simulink subsystem "MotorDriveGearTh"  (R2024b)
settings: Solver=VariableStepAuto  StartTime=0.0  StopTime=10.0  RelTol=1e-3
model mask{max_torque=electricDrive.max_torque, max_power=electricDrive.max_power, Tctc=electricDrive.Tctc, motor_loss_map=electricDrive.motor_loss_map, coolant_channel_D=electricDrive.coolant_channel_D}
  mask prompts: Tctc "Motor torque control time constant(s)"; coolant_channel_D "[m] Coolant jacket channels diameter"
undefined symbols (not defined in the file or in its folder): electricDrive, vehicleThermal
libraries: fl_lib x20, ee_lib x4, SimscapeFluids_lib x2, nesl_utility x2, EmotorLib x1, sdl_lib x1
Description:
  | Motor Drive with Gear (Thermal)
  | 
  | ⚡ Main Features:
  | - Electric motor model coupled with fixed gear
  | - Motor input interface: torque command, battery signals, and control
  | - Includes motor plant with electrical, mechanical, and thermal ports
  | - Coolant jacket for motor thermal management
  | - Inverter thermal dynamics with coolant pipe connection
  | - Gear block transmits torque to axle
  | 
  | 📤 Outputs: Motor Torque, Motor Speed, Electrical Power, Thermal States, Energy
  | 
  | 📌 Use Case: Powertrain simulations with electro-mechanical coupling and thermal effects
settings Model: Creator=jjha  LastModifiedBy=jjha

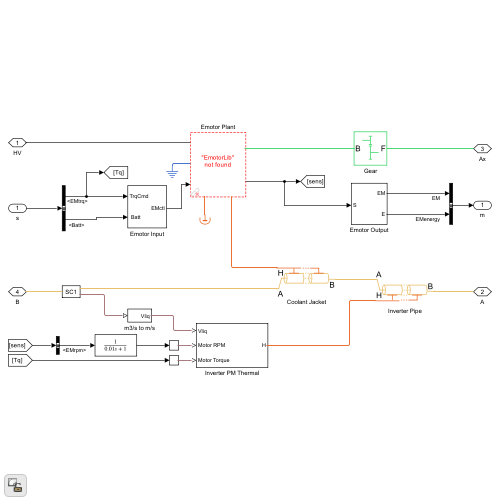
[thumbnail: Simulink's stored preview of the top-level diagram]
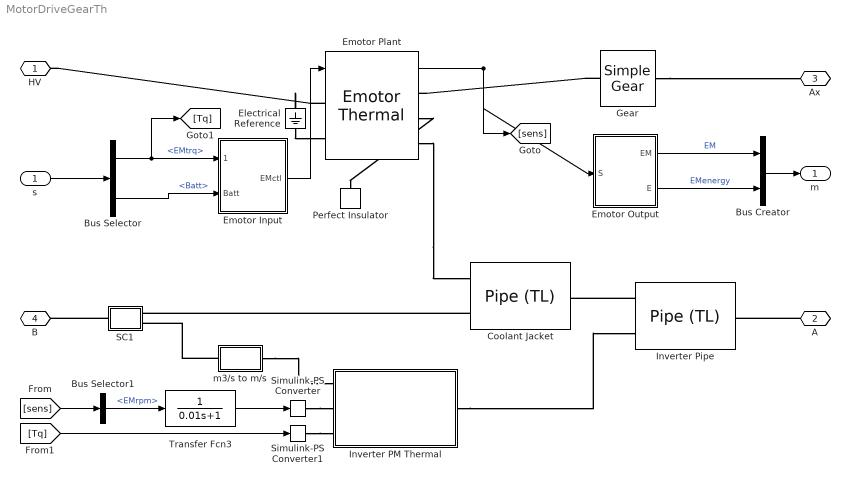
== system MotorDriveGearTh ==
  s : Inport
  Bus Creator : BusCreator  Inputs=2
  Bus Selector : BusSelector  OutputSignals=EMtrq,Batt
  Bus Selector1 : BusSelector  OutputSignals=EMrpm
  Coolant Jacket : SimscapeFluids_lib/Thermal Liquid/Pipes & Fittings/Pipe (TL)  dynamic_compressibility=false  inertia=0  num_segments=1  pipe_length=0.4 m  cross_section_geometry=fluids.thermal_liquid.pipes_fittings.enum.CrossSectionGeometry.Custom  pipe_diameter=0.1 m  pipe_inner_diameter=0.05 m  pipe_outer_diameter=0.1 m  pipe_width=0.1 m  pipe_height=0.1 m  pipe_major_axis=0.1 m  pipe_minor_axis=0.05 m  pipe_side=0.1 m  pipe_angle=30 deg  area=4 * pi * electricDrive.coolant_channel_D^2 / 4 m^2  Dh=electricDrive.coolant_channel_D m  elevation_spec=foundation.enum.constant_variable.constant  elevation_gain=0 m  gravity_spec=foundation.enum.constant_variable.constant  g=9.81 m/s^2  pressure_loss_spec=1  local_pressure_loss_spec=fluids.thermal_liquid.pipes_fittings.enum.LocalLossSpec.AggregateLength  length_add=20 * electricDrive.coolant_channel_D * 4 m  loss_coefficient=0.1  roughness_spec=fluids.thermal_liquid.pipes_fittings.enum.RoughnessSpec.Custom  roughness=1.5e-5 m  Re_friction_TLU=[ 400 1000 1.5e+3 3e+3 4e+3 6e+3 1e+4 2e+4 4e+4 6e+4 1e+5 1e+8 ]  friction_factor_TLU=[ 0.264 0.112 0.07099999999999999 0.0417 0.0387 0.0268 0.025 0.0232 0.0226 0.022 0.0214 0.0214 ]  Re_lam=100  Re_tur=500  shape_factor=64  mdot_nominal=[ 0.1 1 ] kg/s  p_diff_nominal=[ 0.001 0.01 ] MPa  mdot_threshold=1e-6 kg/s  wall_spec=1  vol_expansion_spec=fluids.thermal_liquid.pipes_fittings.enum.VolumeExpansionSpec.Diameter  area_pressure_gain=1e-6 m^2/MPa  static_pressure_TLU=[.1, 1] MPa  area_pressure_gain_TLU=[1e-05, 1.1e-05] m^2  material_behavior_spec=fluids.thermal_liquid.pipes_fittings.enum.PipeMaterialBehavior.Linear  diameter_pressure_gain=1.2e-6 m/MPa  wall_thickness=0.05 m  elastic_modulus=69 GPa  stress_TLU=[276, 310] MPa  strain_TLU=[.004, .02]  stress_assert_action=simscape.enum.assert.action.none  stress_max=400 MPa  poisson_ratio=0.33  wall_time_constant=0.01 s  thermal_expansion=false  alpha_L_wall=24 um/(deltaK*m)  thermal_expansion_Tref=293.15 K  heat_transfer_spec=4  mdot_nominal_heat=[ 0.1 1 ] kg/s  T_in_nominal=[ 293.15 293.15 ] K  T_out_nominal=[ 300 300 ] K  p_in_nominal_heat=[ 0.101325 0.101325 ] MPa  T_wall_nominal=[ 303.15 303.15 ] K  a_coeff=0.3  b_Re_power=0.8  c_Pr_power=0.33  Nu_lam=3.66  Re_Colburn_TLU=[ 100 150 1000 ]  Colburn_factor_TLU=[ 0.019 0.013 0.002 ]  Re_Nu_TLU=[ 100 150 1000 ]  Pr_Nu_TLU=[ 1 10 ]  Nu_TLU=[ 3.72 4.21; 3.75 4.44; 4.21 7.15 ]  p0_vec=vehicleThermal.coolant_p_init MPa  T0_vec=vehicleThermal.coolant_T_init K  mdot0=0.1 kg/s
  Electrical Reference : fl_lib/Electrical/Electrical Elements/Electrical Reference
  Emotor Input : Subsystem
  Emotor Output : Subsystem
  Emotor Plant : EmotorLib/Emotor Thermal  InitTemp=vehicleThermal.coolant_T_init  IronSpHeat=electricDrive.IronSpHeat  CopperSpHeat=electricDrive.CopperSpHeat  IronThConductivity=electricDrive.IronThConductivity  GrossToothMass=electricDrive.MotorThermal.GrossToothMass  WindingMass=electricDrive.MotorThermal.WindingMass  max_torque=electricDrive.max_torque  max_power=electricDrive.max_power  Tctc=electricDrive.Tctc  spMat=electricDrive.motor_loss_map.spMat  tqMat=electricDrive.motor_loss_map.tqMat  lossMat=electricDrive.motor_loss_map.lossMat  StatorBackIronMass=electricDrive.MotorThermal.StatorBackIronMass  StatorRootDia=electricDrive.MotorThermal.StatorRootDia  stator_od=electricDrive.MotorThermal.stator_od  StatorWindingOhArea=electricDrive.MotorThermal.StatorWindingOhArea  Bridgemass=electricDrive.MotorThermal.Bridgemass  rotor_od=electricDrive.MotorThermal.rotor_od  rotorStackLength=electricDrive.MotorThermal.rotorStackLength  RotorBackIronMass=electricDrive.MotorThermal.RotorBackIronMass  RotorAreaER=electricDrive.MotorThermal.RotorAreaER  RotorAreaCyl=electricDrive.MotorThermal.RotorAreaCyl
  Gear : sdl_lib/Gears/Simple Gear  ratio=10/3  rotation_direction=sdl.enum.shaftOutputDirection.same  friction_model=sdl.enum.gear_efficiencies_load.off  T_noload=0.1 N*m  T_nom=5 N*m  efficiency_nom=0.8  efficiency=0.8  temperature_TLU=[280, 300, 320] K  load_TLU=[1, 5, 10] N*m  efficiency_TLU=[.95, .9, .85]  efficiency_TLU2=[.85, .8, .75; .95, .9, .85; .85, .8, .7]  w_thr=0.01 rad/s  pwr_thr=0.001 W  enable_backlash=false  hardstop_model=simscape.enum.hardstop.smooth  backlash_distance=1e-3 mm  r_base=0.1 m  transition=1e-4 mm  backlash_stiffness=1e7 N/m  backlash_damping=1e6 N*s/m  coeff_rest=0  v_tol=0.001 m/s  f_tol=0 N  mu_visc=[0, 0] N*m*s/rad  thermal_mass=50 J/K  temperature_specify=off  temperature_priority=High  temperature=300 K  temperature_nominal_specify=off  temperature_nominal_value=1  temperature_nominal_unit=K  x_backlash_specify=off  x_backlash_priority=None  x_backlash=0 mm  x_backlash_nominal_specify=off  x_backlash_nominal_value=1  x_backlash_nominal_unit=mm  f_hardstop_specify=off  f_hardstop_priority=None  f_hardstop=0 N  f_hardstop_nominal_specify=off  f_hardstop_nominal_value=1  f_hardstop_nominal_unit=N  v_backlash_specify=off  v_backlash_priority=None  v_backlash=0 m/s  v_backlash_nominal_specify=off  v_backlash_nominal_value=1  v_backlash_nominal_unit=m/s
  Inverter PM Thermal : Subsystem
  Inverter Pipe : SimscapeFluids_lib/Thermal Liquid/Pipes & Fittings/Pipe (TL)  dynamic_compressibility=false  inertia=0  num_segments=1  pipe_length=0.4 m  cross_section_geometry=fluids.thermal_liquid.pipes_fittings.enum.CrossSectionGeometry.Custom  pipe_diameter=0.1 m  pipe_inner_diameter=0.05 m  pipe_outer_diameter=0.1 m  pipe_width=0.1 m  pipe_height=0.1 m  pipe_major_axis=0.1 m  pipe_minor_axis=0.05 m  pipe_side=0.1 m  pipe_angle=30 deg  area=4 * pi * electricDrive.coolant_channel_D^2 / 4 m^2  Dh=electricDrive.coolant_channel_D m  elevation_spec=foundation.enum.constant_variable.constant  elevation_gain=0 m  gravity_spec=foundation.enum.constant_variable.constant  g=9.81 m/s^2  pressure_loss_spec=1  local_pressure_loss_spec=fluids.thermal_liquid.pipes_fittings.enum.LocalLossSpec.AggregateLength  length_add=20 * electricDrive.coolant_channel_D * 4 m  loss_coefficient=0.1  roughness_spec=fluids.thermal_liquid.pipes_fittings.enum.RoughnessSpec.Custom  roughness=1.5e-5 m  Re_friction_TLU=[ 400 1000 1.5e+3 3e+3 4e+3 6e+3 1e+4 2e+4 4e+4 6e+4 1e+5 1e+8 ]  friction_factor_TLU=[ 0.264 0.112 0.07099999999999999 0.0417 0.0387 0.0268 0.025 0.0232 0.0226 0.022 0.0214 0.0214 ]  Re_lam=100  Re_tur=500  shape_factor=64  mdot_nominal=[ 0.1 1 ] kg/s  p_diff_nominal=[ 0.001 0.01 ] MPa  mdot_threshold=1e-6 kg/s  wall_spec=1  vol_expansion_spec=fluids.thermal_liquid.pipes_fittings.enum.VolumeExpansionSpec.Diameter  area_pressure_gain=1e-6 m^2/MPa  static_pressure_TLU=[.1, 1] MPa  area_pressure_gain_TLU=[1e-05, 1.1e-05] m^2  material_behavior_spec=fluids.thermal_liquid.pipes_fittings.enum.PipeMaterialBehavior.Linear  diameter_pressure_gain=1.2e-6 m/MPa  wall_thickness=0.05 m  elastic_modulus=69 GPa  stress_TLU=[276, 310] MPa  strain_TLU=[.004, .02]  stress_assert_action=simscape.enum.assert.action.none  stress_max=400 MPa  poisson_ratio=0.33  wall_time_constant=0.01 s  thermal_expansion=false  alpha_L_wall=24 um/(deltaK*m)  thermal_expansion_Tref=293.15 K  heat_transfer_spec=4  mdot_nominal_heat=[ 0.1 1 ] kg/s  T_in_nominal=[ 293.15 293.15 ] K  T_out_nominal=[ 300 300 ] K  p_in_nominal_heat=[ 0.101325 0.101325 ] MPa  T_wall_nominal=[ 303.15 303.15 ] K  a_coeff=0.3  b_Re_power=0.8  c_Pr_power=0.33  Nu_lam=3.66  Re_Colburn_TLU=[ 100 150 1000 ]  Colburn_factor_TLU=[ 0.019 0.013 0.002 ]  Re_Nu_TLU=[ 100 150 1000 ]  Pr_Nu_TLU=[ 1 10 ]  Nu_TLU=[ 3.72 4.21; 3.75 4.44; 4.21 7.15 ]  p0_vec=vehicleThermal.coolant_p_init MPa  T0_vec=vehicleThermal.coolant_T_init K  mdot0=0.1 kg/s
  Perfect Insulator : fl_lib/Thermal/Thermal Elements/Perfect Insulator  T_specify=off  T_priority=None  T=293.15 K  T_nominal_specify=off  T_nominal_value=1  T_nominal_unit=K
  SC1 : Subsystem
      mask Display: disp(get_param(gcb, 'Name'))
  Simulink-PS Converter : nesl_utility/Simulink-PS Converter  PhysicalDomain=network_engine_domain  SubClassName=ps_input  LeftPortType=input  RightPortType=output  PseudoPeriodic=off  Frequencies=[]  NoiseDistribution=none  NoiseParameters=[]  Unit=rpm  AffineConversion=off  FilteringAndDerivatives=provide  SimscapeFilterOrder=1  InputFilterTimeConstant=0.001  UdotUserProvided=0
  Simulink-PS Converter1 : nesl_utility/Simulink-PS Converter  PhysicalDomain=network_engine_domain  SubClassName=ps_input  LeftPortType=input  RightPortType=output  PseudoPeriodic=off  Frequencies=[]  NoiseDistribution=none  NoiseParameters=[]  Unit=N*m  AffineConversion=off  FilteringAndDerivatives=provide  SimscapeFilterOrder=1  InputFilterTimeConstant=0.001  UdotUserProvided=0
  Transfer Fcn3 : TransferFcn  Denominator=[0.01 1]
  m3/s to m/s : Subsystem
  HV : PMIOPort  Side=Left
  A : PMIOPort  Port=2  Side=Left
  Ax : PMIOPort  Port=3  Side=Right
  B : PMIOPort  Port=4  Side=Right
  m : Outport
  wires:
  Bus Selector/1 -> Emotor Input/1(TrqCmd), [Tq]  "<EMtrq>"
  Bus Selector/2 -> Emotor Input/2(" Batt")  "<Batt>"
  Emotor Plant/1 -> [sens], Emotor Output/1(S)
  Emotor Input/1(EMctl) -> Emotor Plant/1
  Bus Creator/1 -> m/1
  Emotor Output/1(EM) -> Bus Creator/1  "EM"
  Emotor Output/2(E) -> Bus Creator/2  "EMenergy"
  s/1 -> Bus Selector/1
  [Tq] -> Simulink-PS Converter1/1
  [sens] -> Bus Selector1/1
  Bus Selector1/1 -> Transfer Fcn3/1  "<EMrpm>"
  Transfer Fcn3/1 -> Simulink-PS Converter/1
  connections:
  Gear/LConn1 -- Emotor Plant/RConn1
  Emotor Plant/LConn1 -- HV/RConn1
  Inverter Pipe/LConn1 -- Coolant Jacket/RConn1
  m3/s to m/s/RConn1 -- Inverter PM Thermal/LConn1
  Simulink-PS Converter1/RConn1 -- Inverter PM Thermal/LConn3
  SC1/LConn1 -- B/RConn1
  Inverter PM Thermal/RConn1 -- Inverter Pipe/LConn2
  Coolant Jacket/LConn1 -- SC1/RConn1
  A/RConn1 -- Inverter Pipe/RConn1
  Emotor Plant/RConn3 -- Coolant Jacket/LConn2
  m3/s to m/s/LConn1 -- SC1/RConn2
  Simulink-PS Converter/RConn1 -- Inverter PM Thermal/LConn2
  Emotor Plant/RConn2 -- Perfect Insulator/LConn1
  Gear/RConn1 -- Ax/RConn1
  Electrical Reference/LConn1 -- Emotor Plant/LConn2

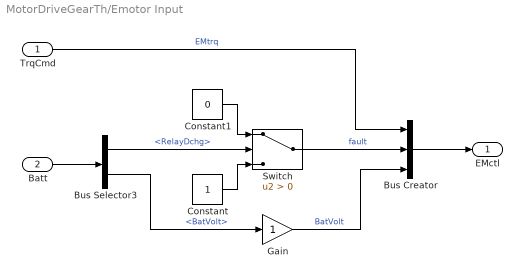
== system MotorDriveGearTh/Emotor Input ==
  TrqCmd : Inport
  " Batt" : Inport  Port=2
  Bus Creator : BusCreator  Inputs=3
  Bus Selector3 : BusSelector  OutputSignals=Relay.RelayDchg,BattSensor.BatVolt
  Constant : Constant
  Constant1 : Constant  Value=0
  Gain : Gain
  Switch : Switch  Criteria=u2 > Threshold  SaturateOnIntegerOverflow=off  InputSameDT=off
  EMctl : Outport
  wires:
  Gain/1 -> Bus Creator/3  "BatVolt"
  Bus Selector3/2 -> Gain/1  "<BatVolt>"
  Bus Creator/1 -> EMctl/1
  " Batt"/1 -> Bus Selector3/1
  Bus Selector3/1 -> Switch/2  "<RelayDchg>"
  Constant/1 -> Switch/3
  Constant1/1 -> Switch/1
  Switch/1 -> Bus Creator/2  "fault"
  TrqCmd/1 -> Bus Creator/1  "EMtrq"

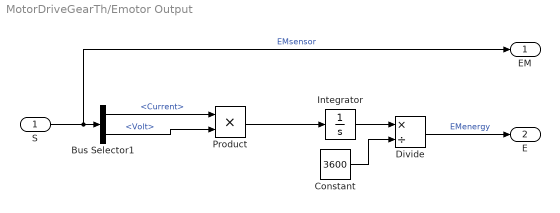
== system MotorDriveGearTh/Emotor Output ==
  S : Inport
  Bus Selector1 : BusSelector  OutputSignals=Current,Volt
  Constant : Constant  Value=3600
  Divide : Product  Inputs=*/
  Integrator : Integrator
  Product : Product
  EM : Outport
  E : Outport  Port=2
  wires:
  Bus Selector1/1 -> Product/1  "<Current>"
  Bus Selector1/2 -> Product/2  "<Volt>"
  S/1 -> Bus Selector1/1, EM/1  "EMsensor"
  Product/1 -> Integrator/1
  Integrator/1 -> Divide/1
  Constant/1 -> Divide/2
  Divide/1 -> E/1  "EMenergy"

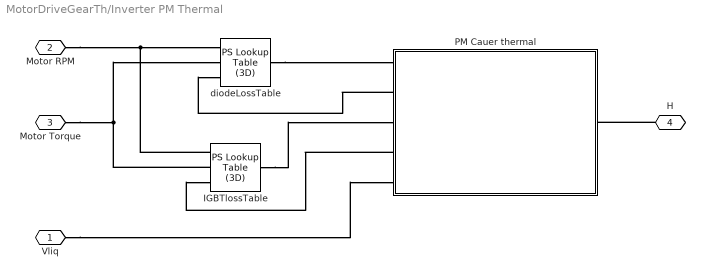
== system MotorDriveGearTh/Inverter PM Thermal ==
  IGBTlossTable : fl_lib/Physical Signals/Lookup Tables/PS Lookup Table (3D)  x1=electricDrive.motor_loss_map.spMat rpm  x2=electricDrive.motor_loss_map.tqMat N*m  x3=[25,125, 175]+273.15 K  f=electricDrive.inverter_loss_map.lossMatIgbt  interp_method=simscape.enum.interpolation.linear  extrap_method=simscape.enum.extrapolation.linear
      settings: InternalSimscapePortConfiguration="{\"Bottom\":[],\"Left\":[{\"id\":\"I1\",\"label\":\"x1\",\"type\":\"input\"},{\"id\":\"I2\",\"label\":\"x2\",\"type\":\"input\"},{\"id\":\"I3\",\"label\":\"x3\",\"type\":\"input\"}],\"Right\":[{\"id\":\"O\",\"label\":\"f\",\"type\":\"output\"}],\"Top\":[]}"
  PM Cauer thermal : Subsystem
  diodeLossTable : fl_lib/Physical Signals/Lookup Tables/PS Lookup Table (3D)  x1=electricDrive.motor_loss_map.spMat rpm  x2=electricDrive.motor_loss_map.tqMat N*m  x3=[25,125, 175]+273.15 K  f=electricDrive.inverter_loss_map.lossMatDiode  interp_method=simscape.enum.interpolation.linear  extrap_method=simscape.enum.extrapolation.linear
      settings: InternalSimscapePortConfiguration="{\"Bottom\":[],\"Left\":[{\"id\":\"I1\",\"label\":\"x1\",\"type\":\"input\"},{\"id\":\"I2\",\"label\":\"x2\",\"type\":\"input\"},{\"id\":\"I3\",\"label\":\"x3\",\"type\":\"input\"}],\"Right\":[{\"id\":\"O\",\"label\":\"f\",\"type\":\"output\"}],\"Top\":[]}"
  Vliq : PMIOPort  Side=Left
  Motor RPM : PMIOPort  Port=2  Side=Left
  Motor Torque : PMIOPort  Port=3  Side=Left
  H : PMIOPort  Port=4  Side=Right
  connections:
  PM Cauer thermal/RConn4 -- IGBTlossTable/LConn3
  PM Cauer thermal/RConn2 -- diodeLossTable/LConn3
  IGBTlossTable/LConn2 -- Motor Torque/RConn1 -- diodeLossTable/LConn2
  IGBTlossTable/LConn1 -- diodeLossTable/LConn1 -- Motor RPM/RConn1
  Vliq/RConn1 -- PM Cauer thermal/RConn5
  diodeLossTable/RConn1 -- PM Cauer thermal/RConn1
  IGBTlossTable/RConn1 -- PM Cauer thermal/RConn3
  H/RConn1 -- PM Cauer thermal/LConn1

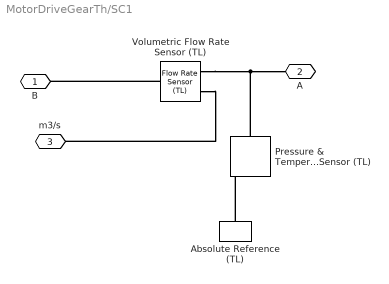
== system MotorDriveGearTh/SC1 ==
  Absolute Reference (TL) : fl_lib/Thermal Liquid/Elements/Absolute Reference (TL)
  Pressure & Temperature Sensor (TL) : fl_lib/Thermal Liquid/Sensors/Pressure & Temperature Sensor (TL)  reference=foundation.enum.MeasurementReference.difference  pressure=true  pressure_spec=foundation.enum.PressureMeasementSpec.Absolute  temperature=true
      settings: InternalSimscapePortConfiguration="{\"Bottom\":[{\"id\":\"T\",\"label\":\"T\",\"type\":\"output\"}],\"Left\":[{\"id\":\"A\",\"label\":\"A\",\"type\":\"foundation.thermal_liquid.thermal_liquid\"}],\"Right\":[{\"id\":\"B\",\"label\":\"B\",\"type\":\"foundation.thermal_liquid.thermal_liquid\"},{\"id\":\"P\",\"label\":\"P\",\"type\":\"output\"}],\"Top\":[]}"
  Volumetric Flow Rate Sensor (TL) : fl_lib/Thermal Liquid/Sensors/Flow Rate Sensor (TL)  mass_flow_measure=false  volumetric_flow_measure=true  energy_flow_measure=false
      settings: InternalSimscapePortConfiguration="{\"Bottom\":[],\"Left\":[{\"id\":\"A\",\"label\":\"A\",\"type\":\"foundation.thermal_liquid.thermal_liquid\"}],\"Right\":[{\"id\":\"B\",\"label\":\"B\",\"type\":\"foundation.thermal_liquid.thermal_liquid\"},{\"id\":\"V\",\"label\":\"V\",\"type\":\"output\"}],\"Top\":[]}"
  B : PMIOPort  Side=Left
  A : PMIOPort  Port=2  Side=Right
  m3/s : PMIOPort  Port=3  Side=Right
  connections:
  Volumetric Flow Rate Sensor (TL)/RConn2 -- m3/s/RConn1
  Absolute Reference (TL)/LConn1 -- Pressure & Temperature Sensor (TL)/RConn1
  Volumetric Flow Rate Sensor (TL)/LConn1 -- B/RConn1
  Volumetric Flow Rate Sensor (TL)/RConn1 -- A/RConn1 -- Pressure & Temperature Sensor (TL)/LConn1

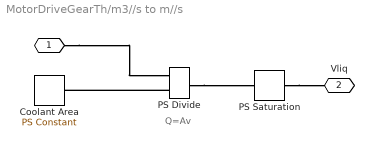
== system MotorDriveGearTh/m3//s to m//s ==
  note: Q=Av
  Coolant Area : fl_lib/Physical Signals/Sources/PS Constant  constant=4 * pi * electricDrive.coolant_channel_D^2 / 4 m^2
  PS Divide : fl_lib/Physical Signals/Functions/PS Divide
  PS Saturation : fl_lib/Physical Signals/Nonlinear Operators/PS Saturation  upper_limit=10 m/s  lower_limit=1e-6 m/s
  "  " : PMIOPort  Side=Left
  Vliq : PMIOPort  Port=2  Side=Right
  connections:
  PS Divide/RConn1 -- PS Saturation/LConn1
  PS Saturation/RConn1 -- Vliq/RConn1
  "  "/RConn1 -- PS Divide/LConn1
  PS Divide/LConn2 -- Coolant Area/RConn1

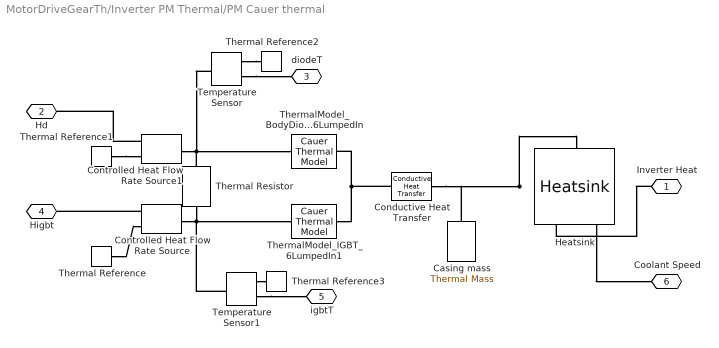
== system MotorDriveGearTh/Inverter PM Thermal/PM Cauer thermal ==
  Casing mass : fl_lib/Thermal/Thermal Elements/Thermal Mass  mass_type=foundation.enum.constant_variable.constant  mass=0.5 kg  sp_heat=447 J/(K*kg)  mass_min=1e-6 kg  num_ports=foundation.enum.numPorts2.one  m_specify=off  m_priority=High  m=1 kg  m_nominal_specify=off  m_nominal_value=1  m_nominal_unit=kg  T_specify=on  T_priority=High  T=vehicleThermal.coolant_T_init K  T_nominal_specify=off  T_nominal_value=1  T_nominal_unit=K  Q_specify=off  Q_priority=None  Q=0 W  Q_nominal_specify=off  Q_nominal_value=1  Q_nominal_unit=W
  Conductive Heat Transfer : fl_lib/Thermal/Thermal Elements/Conductive Heat Transfer  thermal_type=foundation.enum.ConstantVariableTabulated.Constant  wall_geometry=foundation.enum.ConductionWallGeometry.Planar  area=1e-4 m^2  thickness=0.1 m  d_in=0.05 m  d_out=0.1 m  L=1 m  th_cond_min=10 W/(K*m)  th_cond=401 W/(K*m)  th_cond_TLU=[413, 401, 392, 383, 371, 357, 342] W/(K*m)  temp_TLU=[200, 273, 400, 600, 800, 1000, 1200] K  T_specify=off  T_priority=None  T=0 K  T_nominal_specify=off  T_nominal_value=1  T_nominal_unit=K  Q_specify=off  Q_priority=None  Q=0 W  Q_nominal_specify=off  Q_nominal_value=1  Q_nominal_unit=W
  Controlled Heat Flow Rate Source : fl_lib/Thermal/Thermal Sources/Controlled Heat Flow Rate Source
  Controlled Heat Flow Rate Source1 : fl_lib/Thermal/Thermal Sources/Controlled Heat Flow Rate Source
  Heatsink : ee_lib/Passive/Thermal/Heatsink  parameterization=ee.enum.passive.thermal.heatsinkParam.rectangularFin  convection=ee.enum.passive.thermal.heatsinkConvection.specifyFlowSpeed  T_vec_Q=[10, 30, 50, 70, 90] K  v_vec_Q=[0, 1, 2, 3] m/s  Q_TLU1=[6.1, 23.6, 44.5, 67.5, 92.3] W  Q_TLU2=[6.1, 18.8, 22.8, 25.7; 23.6, 61.1, 73, 81.5; 44.5, 106.4, 125.9, 140.1; 67.5, 153.5, 180.7, 200.3; 92.3, 202.1, 236.9, 262] W  T_vec_h=[10, 30, 50, 70, 90] K  v_vec_h=[0, 1, 2, 3] m/s  h_TLU1=[5.4, 7.02, 7.98, 8.68, 9.26] W/(K*m^2)  h_TLU2=[5.4, 17.86, 22.17, 25.41; 7.02, 19.49, 23.8, 27.03; 7.97, 20.44, 24.75, 27.99; 8.68, 21.15, 25.46, 28.69; 9.26, 21.73, 26.04, 29.27] W/(K*m^2)  h_vec=[5, 10, 15, 20, 25, 30] W/(K*m^2)  eff_TLU=[96.97, 94.16, 91.53, 89.08, 86.78, 84.62]  height=electricDrive.HeatsinkParams.Height m  thick=electricDrive.HeatsinkParams.Thick m  depth=electricDrive.HeatsinkParams.Depth m  gap=electricDrive.HeatsinkParams.Gap m  num_fins=electricDrive.HeatsinkParams.NumFins  k_fin=386 W/(K*m)  A_total=0.1171 m^2  nu=2.62e-6 m^2/s  alpha=6.55e-8 m^2/s  k_fluid=0.55 W/(K*m)  beta=5.82e-4 1/K  mass=electricDrive.HeatsinkParams.Mass kg  sp_heat=437 J/(K*kg)  T_hs_specify=on  T_hs_priority=High  T_hs=vehicleThermal.coolant_T_init K  T_hs_nominal_specify=off  T_hs_nominal_value=1  T_hs_nominal_unit=K  Q_A_specify=off  Q_A_priority=None  Q_A=0 W  Q_A_nominal_specify=off  Q_A_nominal_value=1  Q_A_nominal_unit=W  Q_C_specify=off  Q_C_priority=None  Q_C=0 W  Q_C_nominal_specify=off  Q_C_nominal_value=1  Q_C_nominal_unit=W
      settings: InternalSimscapePortConfiguration="{\"Bottom\":[{\"id\":\"C\",\"label\":\"C\",\"type\":\"foundation.thermal.thermal\"}],\"Left\":[{\"id\":\"v\",\"label\":\"v\",\"type\":\"input\"}],\"Right\":[],\"Top\":[{\"id\":\"A\",\"label\":\"A\",\"type\":\"foundation.thermal.thermal\"}]}"
  Temperature Sensor : fl_lib/Thermal/Thermal Sensors/Temperature Sensor  temperature_measure=foundation.enum.MeasurementReference.difference
  Temperature Sensor1 : fl_lib/Thermal/Thermal Sensors/Temperature Sensor  temperature_measure=foundation.enum.MeasurementReference.difference
  Thermal Reference{,1..3} (4 alike) : fl_lib/Thermal/Thermal Elements/Thermal Reference
  Thermal Resistor : ee_lib/Passive/Thermal/Thermal Resistor  R=1e-3 K/W  T_specify=off  T_priority=None  T=0 K  T_nominal_specify=off  T_nominal_value=1  T_nominal_unit=K  Q_specify=off  Q_priority=None  Q=0 W  Q_nominal_specify=off  Q_nominal_value=1  Q_nominal_unit=W
      settings: InternalSimscapePortConfiguration="{\"Bottom\":[],\"Left\":[{\"id\":\"A\",\"label\":\"A\",\"type\":\"foundation.thermal.thermal\"}],\"Right\":[{\"id\":\"B\",\"label\":\"B\",\"type\":\"foundation.thermal.thermal\"}],\"Top\":[]}"
  ThermalModel_BodyDiode_6LumpedIn : ee_lib/Passive/Thermal/Cauer Thermal Model  parameterize_foster=true  resistance_data=1e-3 * [2.6468, 3.8701, 1.2007, .8824] K/W  tau_data=[.0086, .054, .3624, 1.651] s  resistance_data_foster=electricDrive.PMparams.RthDiode K/W  tau_data_foster=electricDrive.PMparams.tauthDiode s  Tvec_specify=on  Tvec_priority=High  Tvec=electricDrive.PMparams.TinitDiode K  Tvec_nominal_specify=off  Tvec_nominal_value=1  Tvec_nominal_unit=K  Q_A_specify=off  Q_A_priority=None  Q_A=0 W  Q_A_nominal_specify=off  Q_A_nominal_value=1  Q_A_nominal_unit=W  Q_B_specify=off  Q_B_priority=None  Q_B=0 W  Q_B_nominal_specify=off  Q_B_nominal_value=1  Q_B_nominal_unit=W
      settings: InternalSimscapePortConfiguration="{\"Bottom\":[],\"Left\":[{\"id\":\"A\",\"label\":\"A\",\"type\":\"foundation.thermal.thermal\"}],\"Right\":[{\"id\":\"B\",\"label\":\"B\",\"type\":\"foundation.thermal.thermal\"}],\"Top\":[]}"
  ThermalModel_IGBT_6LumpedIn1 : ee_lib/Passive/Thermal/Cauer Thermal Model  parameterize_foster=true  resistance_data=1e-3 * [2.6468, 3.8701, 1.2007, .8824] K/W  tau_data=[.0086, .054, .3624, 1.651] s  resistance_data_foster=electricDrive.PMparams.RthIGBT K/W  tau_data_foster=electricDrive.PMparams.tauthIGBT s  Tvec_specify=on  Tvec_priority=High  Tvec=electricDrive.PMparams.TinitIGBT K  Tvec_nominal_specify=off  Tvec_nominal_value=1  Tvec_nominal_unit=K  Q_A_specify=off  Q_A_priority=None  Q_A=0 W  Q_A_nominal_specify=off  Q_A_nominal_value=1  Q_A_nominal_unit=W  Q_B_specify=off  Q_B_priority=None  Q_B=0 W  Q_B_nominal_specify=off  Q_B_nominal_value=1  Q_B_nominal_unit=W
      settings: InternalSimscapePortConfiguration="{\"Bottom\":[],\"Left\":[{\"id\":\"A\",\"label\":\"A\",\"type\":\"foundation.thermal.thermal\"}],\"Right\":[{\"id\":\"B\",\"label\":\"B\",\"type\":\"foundation.thermal.thermal\"}],\"Top\":[]}"
  Inverter Heat : PMIOPort  Side=Left
  Hd : PMIOPort  Port=2  Side=Right
  diodeT : PMIOPort  Port=3  Side=Right
  Higbt : PMIOPort  Port=4  Side=Right
  igbtT : PMIOPort  Port=5  Side=Right
  Coolant Speed : PMIOPort  Port=6  Side=Right
  connections:
  Temperature Sensor/RConn2 -- diodeT/RConn1
  Temperature Sensor/RConn1 -- Thermal Reference2/LConn1
  Temperature Sensor1/RConn2 -- igbtT/RConn1
  Temperature Sensor1/RConn1 -- Thermal Reference3/LConn1
  Heatsink/LConn1 -- Coolant Speed/RConn1
  Inverter Heat/RConn1 -- Heatsink/LConn2
  Controlled Heat Flow Rate Source/RConn1 -- Higbt/RConn1
  Thermal Reference1/LConn1 -- Controlled Heat Flow Rate Source1/RConn2
  Heatsink/RConn1 -- Casing mass/LConn1 -- Conductive Heat Transfer/RConn1
  Conductive Heat Transfer/LConn1 -- ThermalModel_IGBT_6LumpedIn1/RConn1 -- ThermalModel_BodyDiode_6LumpedIn/RConn1
  Controlled Heat Flow Rate Source1/RConn1 -- Hd/RConn1
  Temperature Sensor1/LConn1 -- Thermal Resistor/LConn1 -- ThermalModel_IGBT_6LumpedIn1/LConn1 -- Controlled Heat Flow Rate Source/LConn1
  Thermal Reference/LConn1 -- Controlled Heat Flow Rate Source/RConn2
  Temperature Sensor/LConn1 -- Controlled Heat Flow Rate Source1/LConn1 -- Thermal Resistor/RConn1 -- ThermalModel_BodyDiode_6LumpedIn/LConn1
